simulink model "Linear_Simulation_CTC_Constant_Goal"  (R2020a)
settings: Solver=ode4  StartTime=0.0  StopTime=50  FixedStep=1e-3  RelTol=1e-3
undefined symbols (not defined in the file): Actc, Bctc, Cctc, K, xs0
settings Model: Creator=Pere Giró  LastModifiedBy=Pere Giró

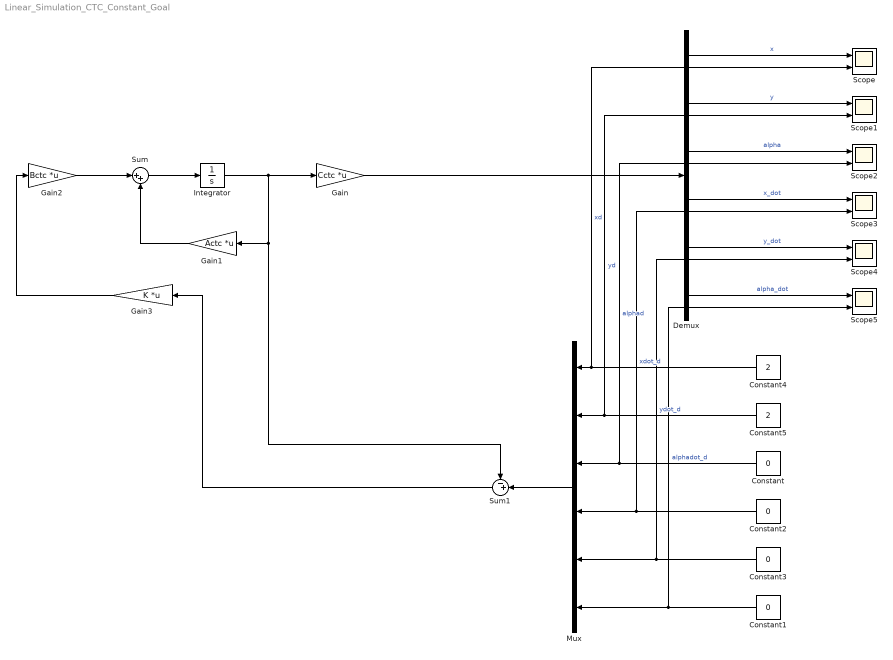
== system Linear_Simulation_CTC_Constant_Goal ==
  Constant{,1..3} (4 alike) : Constant  Value=0
  Constant4 : Constant  Value=2
  Constant5 : Constant  Value=2
  Demux : Demux  Outputs=6
  Gain : Gain  Gain=Cctc  Multiplication=Matrix(K*u)
  Gain1 : Gain  Gain=Actc  Multiplication=Matrix(K*u)
  Gain2 : Gain  Gain=Bctc  Multiplication=Matrix(K*u)
  Gain3 : Gain  Gain=K  Multiplication=Matrix(K*u)
  Integrator : Integrator  InitialCondition=xs0
  Mux : Mux  Inputs=6
  Scope{,1..5} (6 alike) : Scope  NumInputPorts=2
  Sum : Sum  Inputs=|++
  Sum1 : Sum  Inputs=-+|
  wires:
  Gain2/1 -> Sum/1
  Gain1/1 -> Sum/2
  Sum/1 -> Integrator/1
  Integrator/1 -> Gain1/1, Sum1/1, Gain/1
  Gain/1 -> Demux/1
  Demux/1 -> Scope/1  "x"
  Demux/2 -> Scope1/1  "y"
  Demux/3 -> Scope2/1  "alpha"
  Demux/4 -> Scope3/1  "x_dot"
  Demux/5 -> Scope4/1  "y_dot"
  Demux/6 -> Scope5/1  "alpha_dot"
  Gain3/1 -> Gain2/1
  Sum1/1 -> Gain3/1
  Mux/1 -> Sum1/2
  Constant5/1 -> Mux/2, Scope1/2  "yd"
  Constant4/1 -> Scope/2, Mux/1  "xd"
  Constant/1 -> Scope2/2, Mux/3  "alphad"
  Constant1/1 -> Mux/6, Scope5/2  "alphadot_d"
  Constant2/1 -> Mux/4, Scope3/2  "xdot_d"
  Constant3/1 -> Mux/5, Scope4/2  "ydot_d"
